simulink model "newMomentAddTester"  (R2018b)
settings: Solver=VariableStepAuto  StartTime=0.0  StopTime=10  RelTol=1e-3
libraries: filteredPIDController_ul x1
settings Model: Creator=James Reed  LastModifiedBy=jldanie5

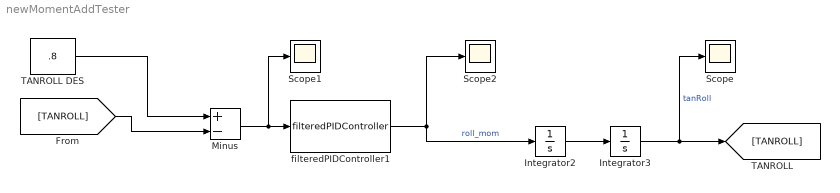
== system newMomentAddTester ==
  Integrator2 : Integrator
  Integrator3 : Integrator
  Minus : Sum  Inputs=+-
  Scope : Scope
  Scope1 : Scope
  Scope2 : Scope
  "TANROLL DES " : Constant  Value=.8
  filteredPIDController1 : filteredPIDController_ul/filteredPIDController  kp=2  ki=0  kd=5  Value=.0000001
  wires:
  "TANROLL DES "/1 -> Minus/1
  filteredPIDController1/1 -> Integrator2/1, Scope2/1  "roll_mom"
  Integrator2/1 -> Integrator3/1
  Integrator3/1 -> Scope/1, [TANROLL]  "tanRoll"
  [TANROLL] -> Minus/2
  Minus/1 -> Scope1/1, filteredPIDController1/1
